simulink model "NM100A_MotVelCtrl"  (R2013b)
settings: Solver=FixedStepDiscrete  SolverMode=SingleTasking  StartTime=0.0  StopTime=1  FixedStep=0.002  RelTol=1e-3
values from neighbouring files (symbols this model uses):
  ARCHGLBPRM_2MILLISEC_SEC_F32 = DataDict.Constant    [NM100A_MotVelCtrl_DataDict.m]
  DERIVTVLPFILTICONLOWRLIM_SEC_F32 = DataDict.Constant    [NM100A_MotVelCtrl_DataDict.m]
  FALSE_CNT_LGC = DataDict.Constant    [NM100A_MotVelCtrl_DataDict.m]
  MOTVELTHDRAMPDWNCMPL_MOTRADPERSEC_F32 = DataDict.Constant    [NM100A_MotVelCtrl_DataDict.m]
  ONEMILLISEC_SEC_F32 = DataDict.Constant    [NM100A_MotVelCtrl_DataDict.m]
  TITHDRAMPDWNCMPL_CNT_U16 = DataDict.Constant    [NM100A_MotVelCtrl_DataDict.m]
  TRUE_CNT_LGC = DataDict.Constant    [NM100A_MotVelCtrl_DataDict.m]
  ZEROMOTVELTAR_MOTRADPERSEC_F32 = DataDict.Constant    [NM100A_MotVelCtrl_DataDict.m]
  ZEROTQCMD_MOTNWTMTR_F32 = DataDict.Constant    [NM100A_MotVelCtrl_DataDict.m]
libraries: NxtrLim x13, simulink x1, NxtrAbslt x1, NxtrMax x1
(part 4 of 4)

== system NM100A_MotVelCtrl/MotVelCtrl/MotVelCtrlPer1/State 3/GetTiSpan100MicroSec32bit/Wrapping ==
  new : Inport
  ref : Inport  Port=2
  Action Port : ActionPort  ActionType=else
  Max Counts : Constant  Value=2^32-1  OutDataTypeStr=uint32
  Subtract1 : Sum  Inputs=+-+
  Out1 : Outport
  wires:
  new/1 -> Subtract1/3
  ref/1 -> Subtract1/2
  Max Counts/1 -> Subtract1/1
  Subtract1/1 -> Out1/1

== system NM100A_MotVelCtrl/MotVelCtrl/MotVelCtrlPer1/State 3/If Action Subsystem/CopyRight2 ==

== system NM100A_MotVelCtrl/MotVelCtrl/MotVelCtrlPer1/State 3/SetManTqCmd/CopyRight2 ==

== system NM100A_MotVelCtrl/MotVelCtrl/MotVelCtrlPer1/State 4/SetManTqCmd/CopyRight2 ==
